simulink model "Simulation"  (R2023b)
settings: Solver=VariableStepAuto  StartTime=0.0  StopTime=tfin  RelTol=1e-3
values from neighbouring files (symbols this model uses):
  Adj = Adj1'    [graph_plot.m]
  G = digraph(Adj)    [graph_plot.m]
undefined symbols (not defined in the file or in its folder): A, B, c, C, F, K, Ko, L1, x0_0, xi_0
libraries: simulink x7
settings Model: Creator=fedpa  LastModifiedBy=fedpa

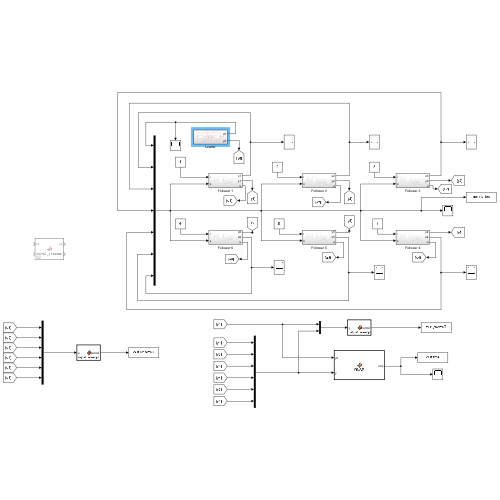
[thumbnail: Simulink's stored preview of the top-level diagram]
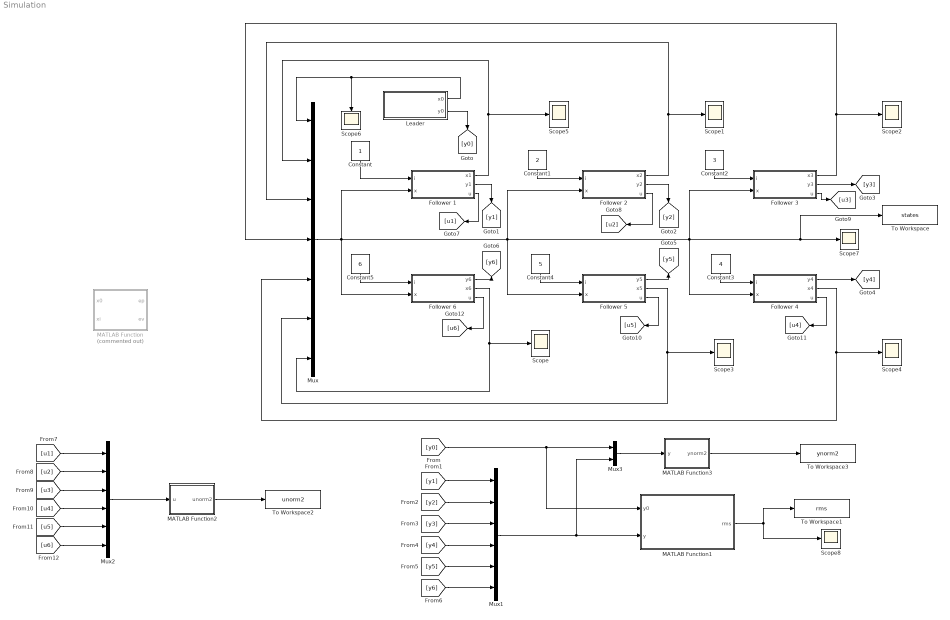
== system Simulation ==
  Constant : Constant
  Constant1 : Constant  Value=2
  Constant2 : Constant  Value=3
  Constant3 : Constant  Value=4
  Constant4 : Constant  Value=5
  Constant5 : Constant  Value=6
  Follower 1 : Subsystem
  Follower 2 : Subsystem
  Follower 3 : Subsystem
  Follower 4 : Subsystem
  Follower 5 : Subsystem
  Follower 6 : Subsystem
  Leader : Subsystem
  MATLAB Function : MATLAB Function  Commented=on  TreatAsAtomicUnit=on
  MATLAB Function1 : MATLAB Function  TreatAsAtomicUnit=on
  MATLAB Function2 : MATLAB Function  TreatAsAtomicUnit=on
  MATLAB Function3 : MATLAB Function  TreatAsAtomicUnit=on
  Mux : Mux  Inputs=7
  Mux1 : Mux  Inputs=6
  Mux2 : Mux  Inputs=6
  Mux3 : Mux  Inputs=2
  Scope{,1..8} (9 alike) : Scope
  To Workspace : ToWorkspace  VariableName=states  SaveFormat=Timeseries  SampleTime=-1
  To Workspace1 : ToWorkspace  VariableName=rms  SaveFormat=Timeseries  SampleTime=-1
  To Workspace2 : ToWorkspace  VariableName=unorm2  SaveFormat=Timeseries  SampleTime=-1
  To Workspace3 : ToWorkspace  VariableName=ynorm2  SaveFormat=Timeseries  SampleTime=-1
  wires:
  Constant3/1 -> Follower 4/1(i)
  Follower 3/1(x3) -> Scope2/1, Mux/4
  Follower 4/2(x4) -> Mux/5, Scope4/1
  Constant4/1 -> Follower 5/1(i)
  Constant5/1 -> Follower 6/1(i)
  Mux/1 -> Follower 1/2(x), Follower 5/2(x), Follower 2/2(x), Follower 4/2(x), Follower 3/2(x), To Workspace/1, Scope7/1, Follower 6/2(x)
  Follower 5/2(x5) -> Mux/6, Scope3/1
  Constant2/1 -> Follower 3/1(i)
  Follower 1/1(x1) -> Mux/2, Scope5/1
  Follower 2/1(x2) -> Mux/3, Scope1/1
  Constant/1 -> Follower 1/1(i)
  Constant1/1 -> Follower 2/1(i)
  Leader/1(x0) -> Mux/1, Scope6/1
  Follower 6/2(x6) -> Mux/7, Scope/1
  [y0] -> Mux3/1, MATLAB Function1/1(y0)
  Leader/2(y0) -> [y0]
  Mux1/1 -> Mux3/2, MATLAB Function1/2(y)
  MATLAB Function1/1(rms) -> To Workspace1/1, Scope8/1
  Follower 1/2(y1) -> [y1]
  Follower 2/2(y2) -> [y2]
  Follower 3/2(y3) -> [y3]
  Follower 6/1(y6) -> [y6]
  Follower 5/1(y5) -> [y5]
  Follower 4/1(y4) -> [y4]
  [y6] -> Mux1/6
  [y5] -> Mux1/5
  [y4] -> Mux1/4
  [y3] -> Mux1/3
  [y2] -> Mux1/2
  [y1] -> Mux1/1
  [u6] -> Mux2/6
  [u5] -> Mux2/5
  [u4] -> Mux2/4
  [u3] -> Mux2/3
  [u2] -> Mux2/2
  [u1] -> Mux2/1
  Follower 1/3(u) -> [u1]
  Follower 2/3(u) -> [u2]
  Follower 3/3(u) -> [u3]
  Follower 4/3(u) -> [u4]
  Follower 5/3(u) -> [u5]
  Follower 6/3(u) -> [u6]
  Mux2/1 -> MATLAB Function2/1(u)
  MATLAB Function2/1(unorm2) -> To Workspace2/1
  Mux3/1 -> MATLAB Function3/1(y)
  MATLAB Function3/1(ynorm2) -> To Workspace3/1

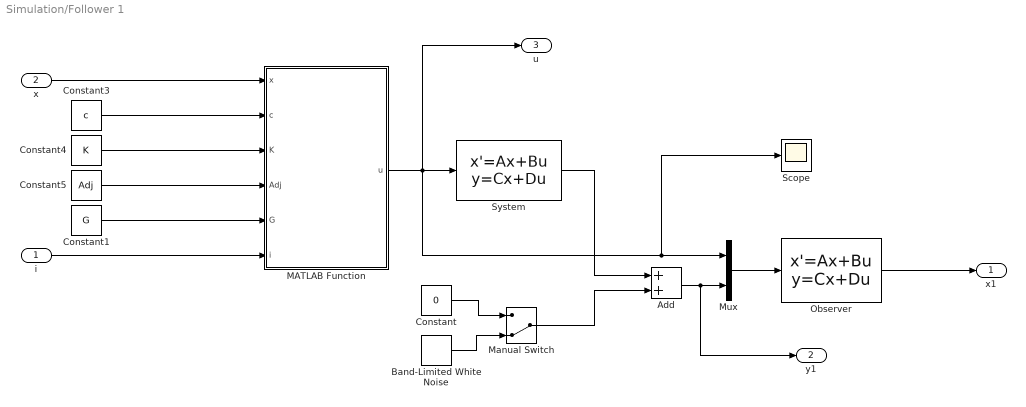
== system Simulation/Follower 1 ==
  i : Inport
  x : Inport  Port=2
  Add : Sum
  Band-Limited White Noise : simulink/Sources/Band-Limited White Noise  Cov=dis  Ts=0.1  seed=[23341]
  Constant : Constant  Value=0
  Constant1 : Constant  Value=G  VectorParams1D=off
  Constant3 : Constant  Value=c
  Constant4 : Constant  Value=K  VectorParams1D=off
  Constant5 : Constant  Value=Adj  VectorParams1D=off
  MATLAB Function : MATLAB Function  TreatAsAtomicUnit=on
  Manual Switch : ManualSwitch  CurrentSetting=0
  Mux : Mux  Inputs=2
  Observer : StateSpace  A=A-B*Ko-c*F*C  B=[B c*F]  C=eye(2)  D=zeros(2,2)  InitialCondition=0
  Scope : Scope
  System : StateSpace  A=A-B*Ko  B=B  C=C  D=0  InitialCondition=xi_0(1:2)
  x1 : Outport
  y1 : Outport  Port=2
  u : Outport  Port=3
  wires:
  MATLAB Function/1(u) -> u/1, Scope/1, Mux/1, System/1
  Mux/1 -> Observer/1
  Observer/1 -> x1/1
  Constant4/1 -> MATLAB Function/3(K)
  i/1 -> MATLAB Function/6(i)
  Constant3/1 -> MATLAB Function/2(c)
  Constant1/1 -> MATLAB Function/5(G)
  Constant5/1 -> MATLAB Function/4(Adj)
  x/1 -> MATLAB Function/1(x)
  Add/1 -> Mux/2, y1/1
  System/1 -> Add/1
  Manual Switch/1 -> Add/2
  Constant/1 -> Manual Switch/1
  Band-Limited White Noise/1 -> Manual Switch/2

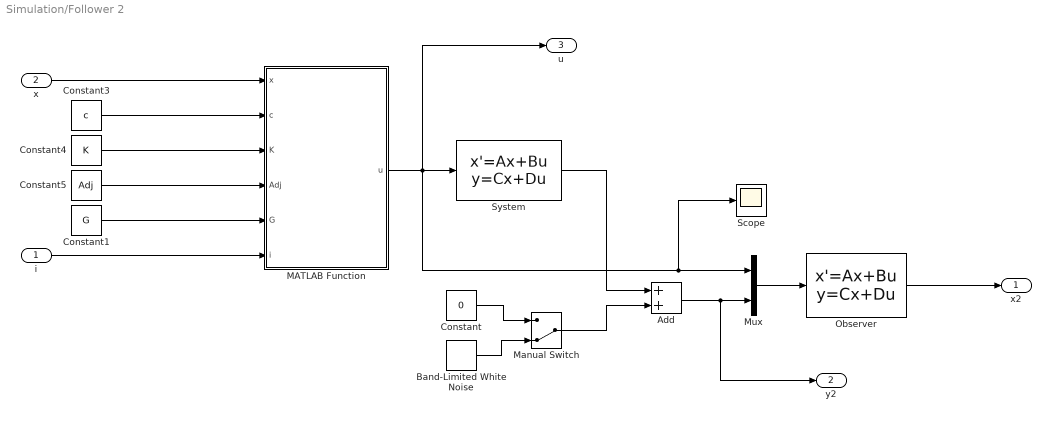
== system Simulation/Follower 2 ==
  i : Inport
  x : Inport  Port=2
  Add : Sum
  Band-Limited White Noise : simulink/Sources/Band-Limited White Noise  Cov=dis  Ts=0.1  seed=[23341]
  Constant : Constant  Value=0
  Constant1 : Constant  Value=G  VectorParams1D=off
  Constant3 : Constant  Value=c
  Constant4 : Constant  Value=K  VectorParams1D=off
  Constant5 : Constant  Value=Adj  VectorParams1D=off
  MATLAB Function : MATLAB Function  TreatAsAtomicUnit=on
  Manual Switch : ManualSwitch  CurrentSetting=0
  Mux : Mux  Inputs=2
  Observer : StateSpace  A=A-B*Ko-c*F*C  B=[B c*F]  C=eye(2)  D=zeros(2,2)  InitialCondition=0
  Scope : Scope
  System : StateSpace  A=A-B*Ko  B=B  C=C  D=0  InitialCondition=xi_0
  x2 : Outport
  y2 : Outport  Port=2
  u : Outport  Port=3
  wires:
  MATLAB Function/1(u) -> u/1, System/1, Scope/1, Mux/1
  Mux/1 -> Observer/1
  Observer/1 -> x2/1
  Constant4/1 -> MATLAB Function/3(K)
  i/1 -> MATLAB Function/6(i)
  Constant3/1 -> MATLAB Function/2(c)
  Constant1/1 -> MATLAB Function/5(G)
  Constant5/1 -> MATLAB Function/4(Adj)
  x/1 -> MATLAB Function/1(x)
  System/1 -> Add/1
  Manual Switch/1 -> Add/2
  Constant/1 -> Manual Switch/1
  Band-Limited White Noise/1 -> Manual Switch/2
  Add/1 -> y2/1, Mux/2

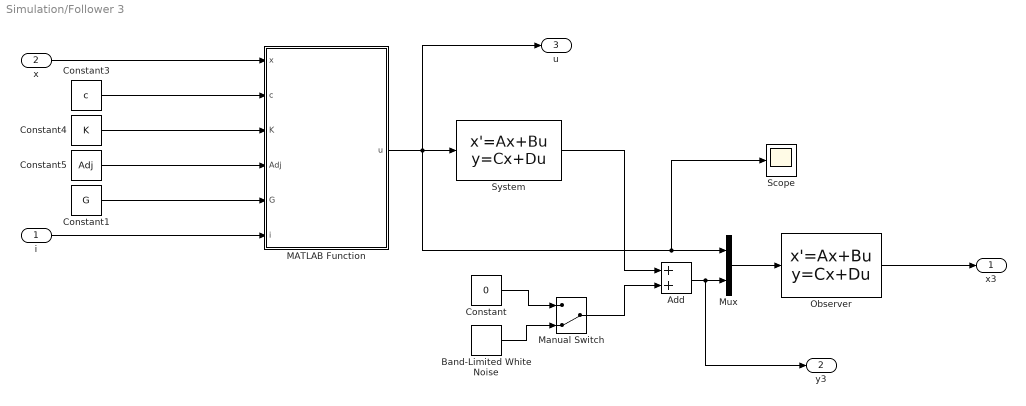
== system Simulation/Follower 3 ==
  i : Inport
  x : Inport  Port=2
  Add : Sum
  Band-Limited White Noise : simulink/Sources/Band-Limited White Noise  Cov=dis  Ts=0.1  seed=[23341]
  Constant : Constant  Value=0
  Constant1 : Constant  Value=G  VectorParams1D=off
  Constant3 : Constant  Value=c
  Constant4 : Constant  Value=K  VectorParams1D=off
  Constant5 : Constant  Value=Adj  VectorParams1D=off
  MATLAB Function : MATLAB Function  TreatAsAtomicUnit=on
  Manual Switch : ManualSwitch  CurrentSetting=0
  Mux : Mux  Inputs=2
  Observer : StateSpace  A=A-B*Ko-c*F*C  B=[B c*F]  C=eye(2)  D=zeros(2,2)  InitialCondition=0
  Scope : Scope
  System : StateSpace  A=A-B*Ko  B=B  C=C  D=0  InitialCondition=xi_0
  x3 : Outport
  y3 : Outport  Port=2
  u : Outport  Port=3
  wires:
  MATLAB Function/1(u) -> u/1, Scope/1, Mux/1, System/1
  Mux/1 -> Observer/1
  Observer/1 -> x3/1
  Constant4/1 -> MATLAB Function/3(K)
  i/1 -> MATLAB Function/6(i)
  Constant3/1 -> MATLAB Function/2(c)
  Constant1/1 -> MATLAB Function/5(G)
  Constant5/1 -> MATLAB Function/4(Adj)
  x/1 -> MATLAB Function/1(x)
  Manual Switch/1 -> Add/2
  System/1 -> Add/1
  Constant/1 -> Manual Switch/1
  Band-Limited White Noise/1 -> Manual Switch/2
  Add/1 -> y3/1, Mux/2

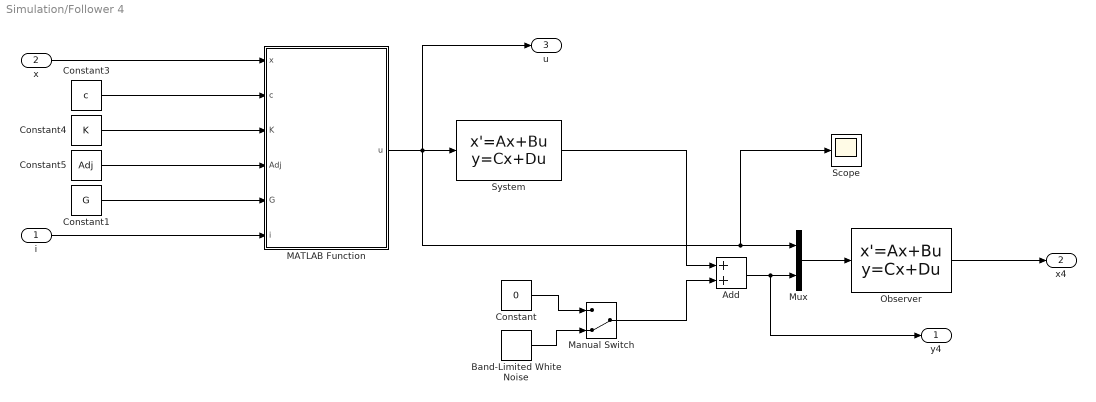
== system Simulation/Follower 4 ==
  i : Inport
  x : Inport  Port=2
  Add : Sum
  Band-Limited White Noise : simulink/Sources/Band-Limited White Noise  Cov=dis  Ts=0.1  seed=[23341]
  Constant : Constant  Value=0
  Constant1 : Constant  Value=G  VectorParams1D=off
  Constant3 : Constant  Value=c
  Constant4 : Constant  Value=K  VectorParams1D=off
  Constant5 : Constant  Value=Adj  VectorParams1D=off
  MATLAB Function : MATLAB Function  TreatAsAtomicUnit=on
  Manual Switch : ManualSwitch  CurrentSetting=0
  Mux : Mux  Inputs=2
  Observer : StateSpace  A=A-B*Ko-c*F*C  B=[B c*F]  C=eye(2)  D=zeros(2,2)  InitialCondition=0
  Scope : Scope
  System : StateSpace  A=A-B*Ko  B=B  C=C  D=0  InitialCondition=xi_0
  y4 : Outport
  x4 : Outport  Port=2
  u : Outport  Port=3
  wires:
  MATLAB Function/1(u) -> u/1, Scope/1, Mux/1, System/1
  Observer/1 -> x4/1
  Constant4/1 -> MATLAB Function/3(K)
  i/1 -> MATLAB Function/6(i)
  Constant3/1 -> MATLAB Function/2(c)
  Constant1/1 -> MATLAB Function/5(G)
  Constant5/1 -> MATLAB Function/4(Adj)
  x/1 -> MATLAB Function/1(x)
  Manual Switch/1 -> Add/2
  Add/1 -> y4/1, Mux/2
  System/1 -> Add/1
  Constant/1 -> Manual Switch/1
  Band-Limited White Noise/1 -> Manual Switch/2
  Mux/1 -> Observer/1

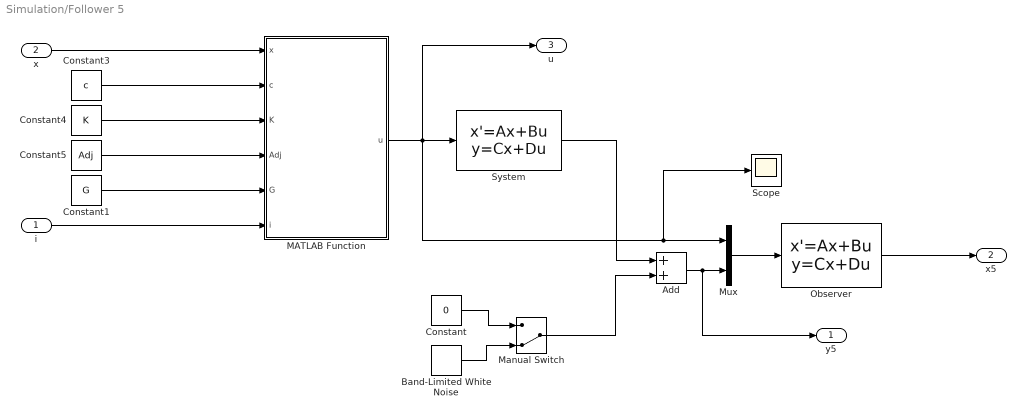
== system Simulation/Follower 5 ==
  i : Inport
  x : Inport  Port=2
  Add : Sum
  Band-Limited White Noise : simulink/Sources/Band-Limited White Noise  Cov=dis  Ts=0.1  seed=[23341]
  Constant : Constant  Value=0
  Constant1 : Constant  Value=G  VectorParams1D=off
  Constant3 : Constant  Value=c
  Constant4 : Constant  Value=K  VectorParams1D=off
  Constant5 : Constant  Value=Adj  VectorParams1D=off
  MATLAB Function : MATLAB Function  TreatAsAtomicUnit=on
  Manual Switch : ManualSwitch  CurrentSetting=0
  Mux : Mux  Inputs=2
  Observer : StateSpace  A=A-B*Ko-c*F*C  B=[B c*F]  C=eye(2)  D=zeros(2,2)  InitialCondition=0
  Scope : Scope
  System : StateSpace  A=A-B*Ko  B=B  C=C  D=0  InitialCondition=xi_0
  y5 : Outport
  x5 : Outport  Port=2
  u : Outport  Port=3
  wires:
  MATLAB Function/1(u) -> u/1, Scope/1, Mux/1, System/1
  Mux/1 -> Observer/1
  Observer/1 -> x5/1
  Constant4/1 -> MATLAB Function/3(K)
  i/1 -> MATLAB Function/6(i)
  Constant3/1 -> MATLAB Function/2(c)
  Constant1/1 -> MATLAB Function/5(G)
  Constant5/1 -> MATLAB Function/4(Adj)
  x/1 -> MATLAB Function/1(x)
  Add/1 -> y5/1, Mux/2
  System/1 -> Add/1
  Constant/1 -> Manual Switch/1
  Band-Limited White Noise/1 -> Manual Switch/2
  Manual Switch/1 -> Add/2

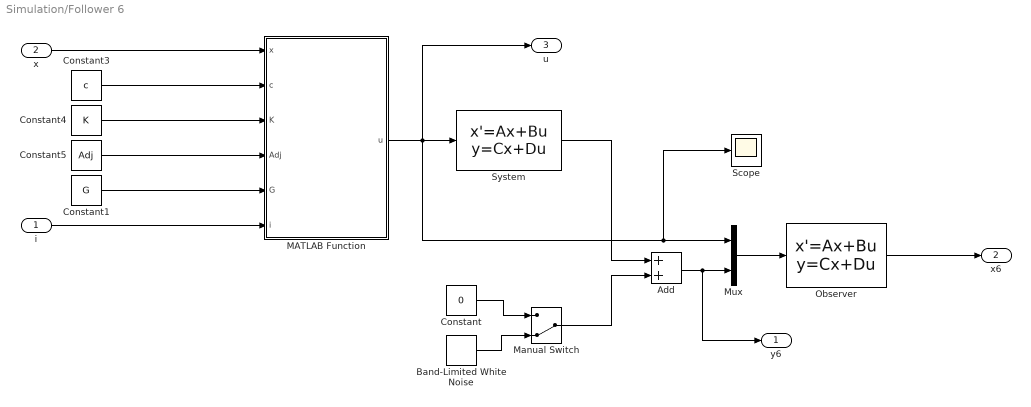
== system Simulation/Follower 6 ==
  i : Inport
  x : Inport  Port=2
  Add : Sum
  Band-Limited White Noise : simulink/Sources/Band-Limited White Noise  Cov=dis  Ts=0.1  seed=[23341]
  Constant : Constant  Value=0
  Constant1 : Constant  Value=G  VectorParams1D=off
  Constant3 : Constant  Value=c
  Constant4 : Constant  Value=K  VectorParams1D=off
  Constant5 : Constant  Value=Adj  VectorParams1D=off
  MATLAB Function : MATLAB Function  TreatAsAtomicUnit=on
  Manual Switch : ManualSwitch  CurrentSetting=0
  Mux : Mux  Inputs=2
  Observer : StateSpace  A=A-B*Ko-c*F*C  B=[B c*F]  C=eye(2)  D=zeros(2,2)  InitialCondition=0
  Scope : Scope
  System : StateSpace  A=A-B*Ko  B=B  C=C  D=0  InitialCondition=xi_0
  y6 : Outport
  x6 : Outport  Port=2
  u : Outport  Port=3
  wires:
  MATLAB Function/1(u) -> u/1, Scope/1, Mux/1, System/1
  Mux/1 -> Observer/1
  Observer/1 -> x6/1
  Constant4/1 -> MATLAB Function/3(K)
  i/1 -> MATLAB Function/6(i)
  Constant3/1 -> MATLAB Function/2(c)
  Constant1/1 -> MATLAB Function/5(G)
  Constant5/1 -> MATLAB Function/4(Adj)
  x/1 -> MATLAB Function/1(x)
  Manual Switch/1 -> Add/2
  Add/1 -> y6/1, Mux/2
  System/1 -> Add/1
  Constant/1 -> Manual Switch/1
  Band-Limited White Noise/1 -> Manual Switch/2

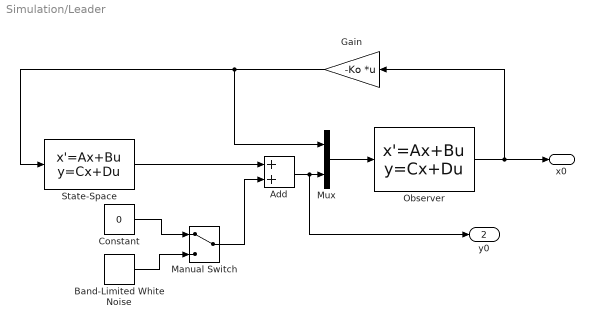
== system Simulation/Leader ==
  Add : Sum
  Band-Limited White Noise : simulink/Sources/Band-Limited White Noise  Cov=dis  Ts=0.1  seed=[23341]
  Constant : Constant  Value=0
  Gain : Gain  Gain=-Ko  Multiplication=Matrix(K*u)
  Manual Switch : ManualSwitch
  Mux : Mux  Inputs=2
  Observer : StateSpace  A=A-L1*C  B=[B L1]  C=eye(2)  D=zeros(2,2)  InitialCondition=0
  State-Space : StateSpace  A=A  B=B  C=C  D=0  InitialCondition=x0_0
  x0 : Outport
  y0 : Outport  Port=2
  wires:
  Gain/1 -> State-Space/1, Mux/1
  Observer/1 -> Gain/1, x0/1
  Mux/1 -> Observer/1
  State-Space/1 -> Add/1
  Add/1 -> y0/1, Mux/2
  Manual Switch/1 -> Add/2
  Band-Limited White Noise/1 -> Manual Switch/2
  Constant/1 -> Manual Switch/1

== matlab function Simulation/MATLAB Function2 ==
  data: u input; unorm2 output
function unorm2 = input_energy(u)
    unorm2 = 0;
    for i=1:6
        unorm2 = unorm2 + norm(u(i))^2;
    end
    unorm2 = unorm2/6;
end

== matlab function Simulation/MATLAB Function3 ==
  data: y input; ynorm2 output
function ynorm2 = output_energy(y)
    ynorm2 = 0;
    for i=1:7
        ynorm2 = ynorm2+norm(y(i))^2;
    end
    ynorm2 = ynorm2/7;

end

== matlab function Simulation/Follower 2/MATLAB Function ==
  data: x input; u output; c input; K input; Adj input; G input; i input
function u = controller(x, c, K, Adj, G, i)
    epsi = zeros(2,1);
    sub = G(i,i)*(x(1:2)-x(i*2+1:i*2+2));
    for j = 1:6
        epsi = epsi + Adj(i,j)*(x(j*2+1:j*2+2)-x(i*2+1:i*2+2));
    end
    epsi = epsi+sub;
    
    u = c*K*epsi;
end

== matlab function Simulation/Follower 1/MATLAB Function ==
  data: x input; u output; c input; K input; Adj input; G input; i input
function u = controller(x, c, K, Adj, G, i)
    epsi = zeros(2,1);
    sub = G(i,i)*(x(1:2)-x(i*2+1:i*2+2));
    for j = 1:6
        epsi = epsi + Adj(i,j)*(x(j*2+1:j*2+2)-x(i*2+1:i*2+2));
    end
    epsi = epsi+sub;
    
    u = c*K*epsi;
end

== matlab function Simulation/Follower 3/MATLAB Function ==
  data: x input; u output; c input; K input; Adj input; G input; i input
function u = controller(x, c, K, Adj, G, i)
    epsi = zeros(2,1);
    sub = G(i,i)*(x(1:2)-x(i*2+1:i*2+2));
    for j = 1:6
        epsi = epsi + Adj(i,j)*(x(j*2+1:j*2+2)-x(i*2+1:i*2+2));
    end
    epsi = epsi+sub;
    
    u = c*K*epsi;
end

== matlab function Simulation/Follower 4/MATLAB Function ==
  data: x input; u output; c input; K input; Adj input; G input; i input
function u = controller(x, c, K, Adj, G, i)
    epsi = zeros(2,1);
    sub = G(i,i)*(x(1:2)-x(i*2+1:i*2+2));
    for j = 1:6
        epsi = epsi + Adj(i,j)*(x(j*2+1:j*2+2)-x(i*2+1:i*2+2));
    end
    epsi = epsi+sub;
    
    u = c*K*epsi;
end

== matlab function Simulation/Follower 5/MATLAB Function ==
  data: x input; u output; c input; K input; Adj input; G input; i input
function u = controller(x, c, K, Adj, G, i)
    epsi = zeros(2,1);
    sub = G(i,i)*(x(1:2)-x(i*2+1:i*2+2));
    for j = 1:6
        epsi = epsi + Adj(i,j)*(x(j*2+1:j*2+2)-x(i*2+1:i*2+2));
    end
    epsi = epsi+sub;
    
    u = c*K*epsi;
end

== matlab function Simulation/Follower 6/MATLAB Function ==
  data: x input; u output; c input; K input; Adj input; G input; i input
function u = controller(x, c, K, Adj, G, i)
    epsi = zeros(2,1);
    sub = G(i,i)*(x(1:2)-x(i*2+1:i*2+2));
    for j = 1:6
        epsi = epsi + Adj(i,j)*(x(j*2+1:j*2+2)-x(i*2+1:i*2+2));
    end
    epsi = epsi+sub;
    
    u = c*K*epsi;
end

== matlab function Simulation/MATLAB Function ==
  data: x0 input; ep output; xi input; ev output
function [ep, ev] = norm2_distance(x0, xi)
    ep = norm(x0(1)-xi(1));
    ev = norm(x0(2)-xi(2));
end

== matlab function Simulation/MATLAB Function1 ==
  data: y0 input; rms output; y input
function rms = RMSE(y0, y)
    mid = 0;
    n = 6;
    for i=1:n
        mid = mid + norm(y0-y(i))^2;
    end
    rms = sqrt(mid/n);
end
